simulink model "SporadicImpulse_6DOF"  (R2019a)
settings: Solver=VariableStepAuto  StartTime=0.0  StopTime=40  RelTol=1e-3
InitFcn:
  | Sporadic_Impulse_6DOF_init
values from neighbouring files (symbols this model uses):
  alpha_0 = 0    [Sporadic_Impulse_3DOF_init.m]    (also in Sporadic_Impulse_6DOF_init.m)
  beta_0 = 0    [Sporadic_Impulse_6DOF_init.m]
  g = 9.81    [Sporadic_Impulse_3DOF_init.m]    (also in Sporadic_Impulse_6DOF_init.m)
  gamma_0 = pi/2-deg2rad(6)    [Sporadic_Impulse_3DOF_init.m]    (also in Sporadic_Impulse_6DOF_init.m)
  m_0 = 40    [Sporadic_Impulse_3DOF_init.m]    (also in Sporadic_Impulse_6DOF_init.m)
  V_0 = 0.1    [Sporadic_Impulse_3DOF_init.m]    (also in Sporadic_Impulse_6DOF_init.m)
undefined symbols (not defined in the file or in its folder): F, Light, MIL
libraries: simulink_extras x4, aerolibwind2 x2, aerolibasang x1, aerolibatmos2 x1, vrlib x1, aerolib6dof2 x1, aerolibtransform2 x1
settings Model: Creator=Devansh  LastModifiedBy=Devansh

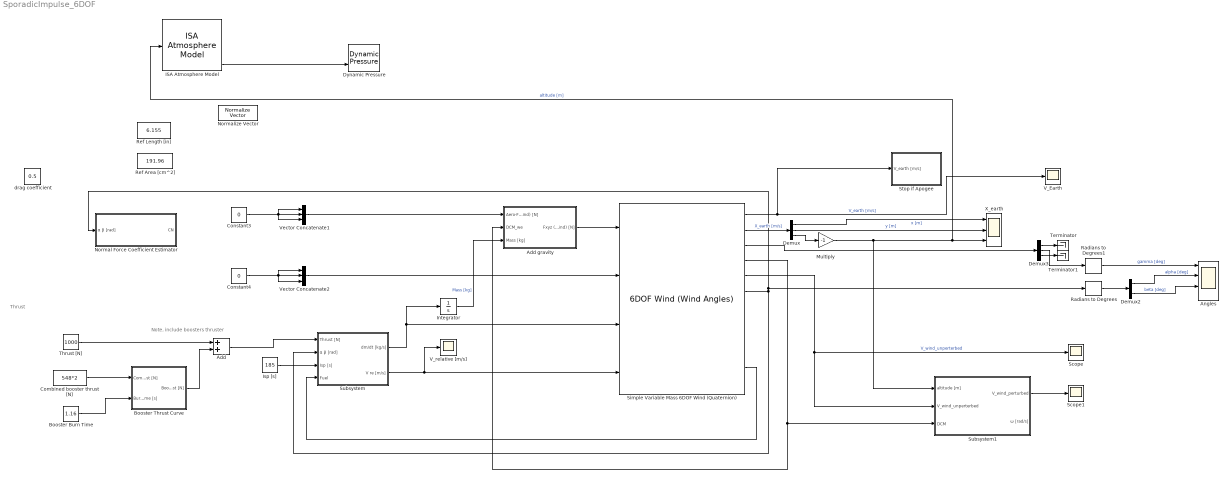
== system SporadicImpulse_6DOF ==
  note: Thrust
  note: Note, include boosters thruster
  Add : Sum
  Add gravity : Subsystem
  Angles : Scope  NumInputPorts=4
  Booster Burn Time : Constant  Value=1.16
  Booster Thrust Curve : Subsystem
  Combined booster thrust [N] : Constant  Value=548*2
  Constant3 : Constant  Value=0
  Constant4 : Constant  Value=0
  Demux : Demux  Outputs=3
  Demux2 : Demux  Outputs=2
  Demux3 : Demux  Outputs=3
  Dynamic Pressure : aerolibasang/Dynamic Pressure
  ISA Atmosphere Model : aerolibatmos2/ISA Atmosphere Model  custom=on  g=9.80665  gamma=1.4  R=287.0531  L=0.0065  h_trop=11000  h_strat=20000  rho0=1.225  P0=101325  T0=288.15  h0=0
      settings: SourceProductName=Aerospace Blockset
  Integrator : Integrator  InitialCondition=m_0
  Isp [s] : Constant  Value=185
  Multiply : Gain  Gain=-1
  Normal Force Coefficient Estimator : Subsystem
  Normalize Vector : vrlib/Utilities/Normalize Vector  maxzero=0
      settings: SourceProductName=Simulink
  Radians to Degrees : simulink_extras/Transformations/Radians to Degrees
  Radians to Degrees1 : simulink_extras/Transformations/Radians to Degrees
  Ref Area [cm^2] : Constant  Value=191.96
  Ref Length [in] : Constant  Value=6.155
  Scope : Scope
  Scope1 : Scope
  Simple Variable Mass 6DOF Wind (Quaternion) : aerolib6dof2/6DOF Wind (Wind Angles)  units=Metric (MKS)  mtype=Simple Variable  rep=Quaternion  xme_0=[0 0 0]  Vm_0=[V_0 alpha_0 beta_0]  wind_0=[0 gamma_0 0]  pm_0=[0 0 0]  mass_0=m_0  mass_e=m_dry  mass_f=m_0  inertia=eye(3)  inertia_e=I_dry  inertia_f=I_0  vre_flag=on  abi_flag=on  xme_statename=''  Vm_statename=''  alpha_statename=''  beta_statename=''  wind_statename=''  quat_statename=''  pm_statename=''  mass_statename=''
      settings: SourceProductName=Aerospace Blockset  SourceProductBaseCode=AE
  Stop if Apogee : Subsystem
  Subsystem : Subsystem
  Subsystem1 : Subsystem
  Terminator : Terminator
  Terminator1 : Terminator
  Thrust [N] : Constant  Value=1000
  V_Earth : Scope
  V_relative [m/s] : Scope
  Vector Concatenate1 : Concatenate  NumInputs=3
  Vector Concatenate2 : Concatenate  NumInputs=3
  X_earth : Scope  NumInputPorts=3
  drag coefficient : Constant  Value=0.5
  wires:
  Constant3/1 -> Vector Concatenate1/3, Vector Concatenate1/1, Vector Concatenate1/2
  Constant4/1 -> Vector Concatenate2/3, Vector Concatenate2/1, Vector Concatenate2/2
  Vector Concatenate2/1 -> Simple Variable Mass 6DOF Wind (Quaternion)/2
  Isp [s]/1 -> Subsystem/3(Isp [s])
  Vector Concatenate1/1 -> Add gravity/1(Aero-Forces (Wind) [N])
  Simple Variable Mass 6DOF Wind (Quaternion)/4 -> Add gravity/2(DCM_we), Subsystem1/3(DCM)
  Integrator/1 -> Add gravity/3(Mass [kg])  "Mass [kg]"
  Add gravity/1(Fxyz (Wind) [N]) -> Simple Variable Mass 6DOF Wind (Quaternion)/1
  Subsystem/1(dm/dt [kg/s]) -> Simple Variable Mass 6DOF Wind (Quaternion)/3, Integrator/1
  Simple Variable Mass 6DOF Wind (Quaternion)/11 -> Subsystem/4(Fuel)
  Simple Variable Mass 6DOF Wind (Quaternion)/1 -> Stop if Apogee/1(V_earth [m/s]), V_Earth/1  "V_earth [m/s]"
  Subsystem/2(V re [m/s]) -> Simple Variable Mass 6DOF Wind (Quaternion)/4, V_relative [m/s]/1
  Simple Variable Mass 6DOF Wind (Quaternion)/2 -> Demux/1  "X_earth [m/s]"
  Demux/3 -> Multiply/1
  Demux/1 -> X_earth/1  "x [m]"
  Demux/2 -> X_earth/2  "y [m]"
  Multiply/1 -> Subsystem1/1(altitude [m]), ISA Atmosphere Model/1, X_earth/3  "altitude [m]"
  Radians to Degrees/1 -> Demux2/1
  Demux2/1 -> Angles/2  "alpha [deg]"
  Demux2/2 -> Angles/3  "beta [deg]"
  Simple Variable Mass 6DOF Wind (Quaternion)/3 -> Demux3/1
  Demux3/2 -> Radians to Degrees1/1
  Thrust [N]/1 -> Add/1
  Add/1 -> Subsystem/1(Thrust [N])
  Combined booster thrust [N]/1 -> Booster Thrust Curve/1(Combined Thrust [N])
  Booster Burn Time/1 -> Booster Thrust Curve/2(Burn Time [s])
  Booster Thrust Curve/1(Booster Thrust [N]) -> Add/2
  Simple Variable Mass 6DOF Wind (Quaternion)/5 -> Scope/1, Subsystem1/2(V_wind_unperterbed)  "V_wind_unperterbed"
  Simple Variable Mass 6DOF Wind (Quaternion)/6 -> Radians to Degrees/1, Normal Force Coefficient Estimator/1(α β [rad]), Subsystem/2(α β [rad])
  ISA Atmosphere Model/4 -> Dynamic Pressure/2
  Demux3/1 -> Terminator/1
  Demux3/3 -> Terminator1/1
  Radians to Degrees1/1 -> Angles/1  "gamma [deg]"
  Subsystem1/1(V_wind_perturbed) -> Scope1/1

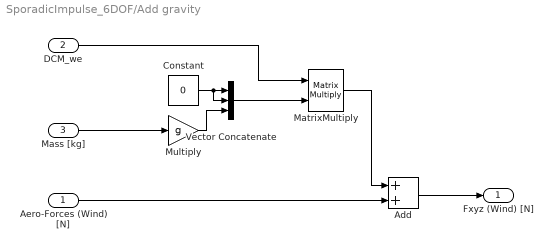
== system SporadicImpulse_6DOF/Add gravity ==
  Aero-Forces (Wind) [N] : Inport
  DCM_we : Inport  Port=2
  Mass [kg] : Inport  Port=3
  Add : Sum
  Constant : Constant  Value=0
  MatrixMultiply : Product  Multiplication=Matrix(*)
  Multiply : Gain  Gain=g
  Vector Concatenate : Concatenate  NumInputs=3
  Fxyz (Wind) [N] : Outport
  wires:
  Aero-Forces (Wind) [N]/1 -> Add/2
  MatrixMultiply/1 -> Add/1
  DCM_we/1 -> MatrixMultiply/1
  Mass [kg]/1 -> Multiply/1
  Multiply/1 -> Vector Concatenate/3
  Constant/1 -> Vector Concatenate/1, Vector Concatenate/2
  Vector Concatenate/1 -> MatrixMultiply/2
  Add/1 -> Fxyz (Wind) [N]/1

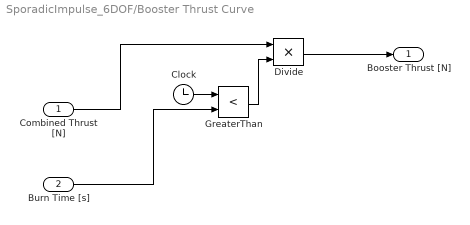
== system SporadicImpulse_6DOF/Booster Thrust Curve ==
  Combined Thrust [N] : Inport
  Burn Time [s] : Inport  Port=2
  Clock : Clock
  Divide : Product  Inputs=**
  GreaterThan : RelationalOperator  Operator=<  OutDataTypeStr=boolean  RndMeth=Simplest
  Booster Thrust [N] : Outport
  wires:
  Combined Thrust [N]/1 -> Divide/1
  Clock/1 -> GreaterThan/1
  Divide/1 -> Booster Thrust [N]/1
  Burn Time [s]/1 -> GreaterThan/2
  GreaterThan/1 -> Divide/2

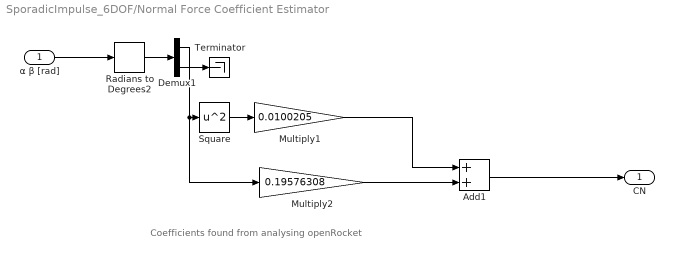
== system SporadicImpulse_6DOF/Normal Force Coefficient Estimator ==
  note: Coefficients found from analysing openRocket
  α β [rad] : Inport
  Add1 : Sum
  Demux1 : Demux  Outputs=2
  Multiply1 : Gain  Gain=0.0100205
  Multiply2 : Gain  Gain=0.19576308
  Radians to Degrees2 : simulink_extras/Transformations/Radians to Degrees
  Square : Math  Operator=square  SaturateOnIntegerOverflow=on
  Terminator : Terminator
  CN : Outport
  wires:
  Add1/1 -> CN/1
  α β [rad]/1 -> Radians to Degrees2/1
  Radians to Degrees2/1 -> Demux1/1
  Demux1/1 -> Multiply2/1, Square/1
  Demux1/2 -> Terminator/1
  Square/1 -> Multiply1/1
  Multiply1/1 -> Add1/1
  Multiply2/1 -> Add1/2

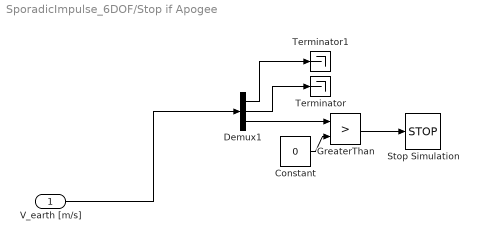
== system SporadicImpulse_6DOF/Stop if Apogee ==
  V_earth [m/s] : Inport
  Constant : Constant  Value=0
  Demux1 : Demux  Outputs=3
  GreaterThan : RelationalOperator  Operator=>  OutDataTypeStr=boolean  RndMeth=Simplest
  Stop Simulation : Stop
  Terminator : Terminator
  Terminator1 : Terminator
  wires:
  Demux1/1 -> Terminator1/1
  Constant/1 -> GreaterThan/2
  Demux1/2 -> Terminator/1
  Demux1/3 -> GreaterThan/1
  V_earth [m/s]/1 -> Demux1/1
  GreaterThan/1 -> Stop Simulation/1

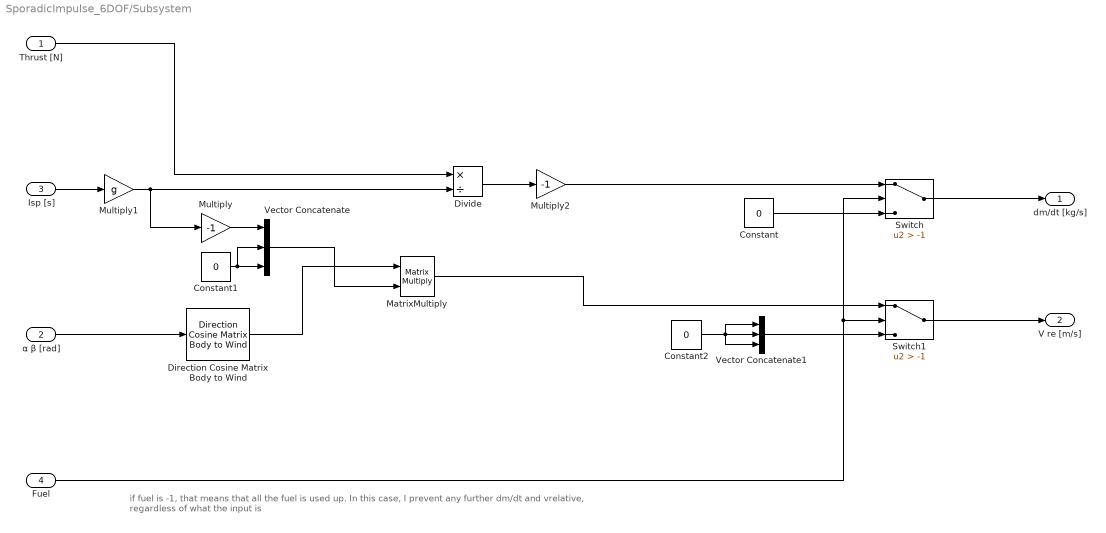
== system SporadicImpulse_6DOF/Subsystem ==
  note: if fuel is -1, that means that all the fuel is used up. In this case, I prevent any further dm/dt and vrelative, regardless of what the input is
  Thrust [N] : Inport
  α β [rad] : Inport  Port=2
  Isp [s] : Inport  Port=3
  Fuel : Inport  Port=4
  Constant : Constant  Value=0
  Constant1 : Constant  Value=0
  Constant2 : Constant  Value=0
  Direction Cosine Matrix Body to Wind : aerolibtransform2/Direction Cosine Matrix Body to Wind
      settings: SourceProductName=Aerospace Blockset  SourceProductBaseCode=AE
  Divide : Product  Inputs=*/
  MatrixMultiply : Product  Multiplication=Matrix(*)
  Multiply : Gain  Gain=-1
  Multiply1 : Gain  Gain=g
  Multiply2 : Gain  Gain=-1
  Switch : Switch  Criteria=u2 > Threshold  Threshold=-1
  Switch1 : Switch  Criteria=u2 > Threshold  Threshold=-1
  Vector Concatenate : Concatenate  NumInputs=3
  Vector Concatenate1 : Concatenate  NumInputs=3
  dm/dt [kg/s] : Outport
  V re [m/s] : Outport  Port=2
  wires:
  α β [rad]/1 -> Direction Cosine Matrix Body to Wind/1
  Divide/1 -> Multiply2/1
  Multiply/1 -> Vector Concatenate/1
  Isp [s]/1 -> Multiply1/1
  Direction Cosine Matrix Body to Wind/1 -> MatrixMultiply/1
  Constant1/1 -> Vector Concatenate/2, Vector Concatenate/3
  Vector Concatenate/1 -> MatrixMultiply/2
  Thrust [N]/1 -> Divide/1
  Multiply1/1 -> Multiply/1, Divide/2
  Fuel/1 -> Switch1/2, Switch/2
  Switch/1 -> dm/dt [kg/s]/1
  Multiply2/1 -> Switch/1
  Constant/1 -> Switch/3
  Switch1/1 -> V re [m/s]/1
  MatrixMultiply/1 -> Switch1/1
  Constant2/1 -> Vector Concatenate1/3, Vector Concatenate1/2, Vector Concatenate1/1
  Vector Concatenate1/1 -> Switch1/3

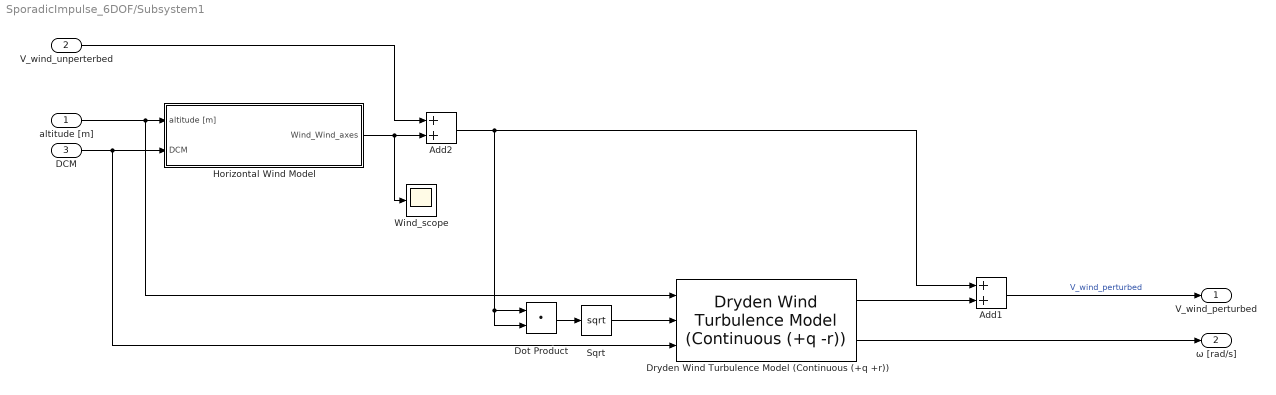
== system SporadicImpulse_6DOF/Subsystem1 ==
  altitude [m] : Inport
  V_wind_unperterbed : Inport  Port=2
  DCM : Inport  Port=3
  Add1 : Sum
  Add2 : Sum
  Dot Product : DotProduct  InputSameDT=on  OutDataTypeStr=Inherit: Inherit via internal rule
  Dryden Wind Turbulence Model (Continuous (+q +r)) : aerolibwind2/Dryden Wind Turbulence Model  (Continuous (+q -r))  units=Metric (MKS)  spec=MIL-F-8785C  model=Continuous Dryden (+q -r)  W20=10  Wdeg=0  TurbProb=10^-2 - Light  L_high=533.4  Wingspan=4  ts=0.1  Seed=[23341 23342 23343 23344]  T_on=on
      settings: SourceProductName=Aerospace Blockset
  Horizontal Wind Model : Subsystem
  Sqrt : Sqrt  SaturateOnIntegerOverflow=on
  Wind_scope : Scope
  V_wind_perturbed : Outport
  ω [rad/s] : Outport  Port=2
  wires:
  Add1/1 -> V_wind_perturbed/1  "V_wind_perturbed"
  V_wind_unperterbed/1 -> Add2/1
  DCM/1 -> Dryden Wind Turbulence Model (Continuous (+q +r))/3, Horizontal Wind Model/2(DCM)
  Dryden Wind Turbulence Model (Continuous (+q +r))/1 -> Add1/2
  Dryden Wind Turbulence Model (Continuous (+q +r))/2 -> ω [rad/s]/1
  altitude [m]/1 -> Dryden Wind Turbulence Model (Continuous (+q +r))/1, Horizontal Wind Model/1(altitude [m])
  Horizontal Wind Model/1(Wind_Wind_axes) -> Wind_scope/1, Add2/2
  Add2/1 -> Dot Product/2, Dot Product/1, Add1/1
  Dot Product/1 -> Sqrt/1
  Sqrt/1 -> Dryden Wind Turbulence Model (Continuous (+q +r))/2

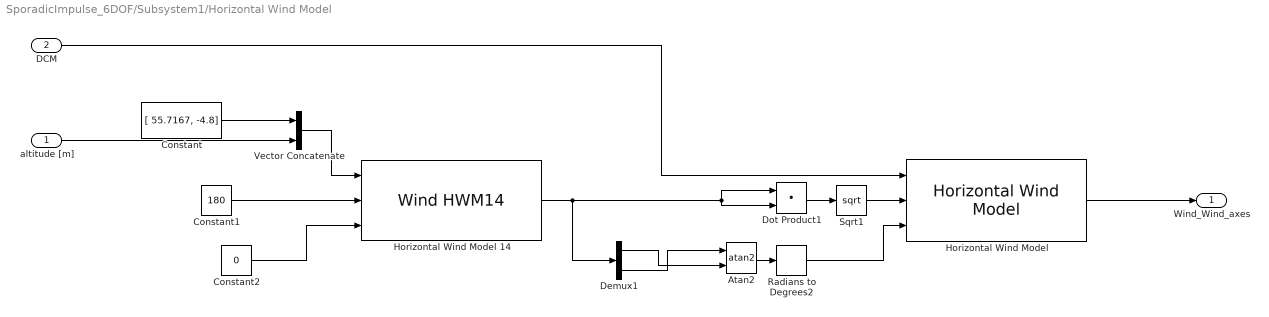
== system SporadicImpulse_6DOF/Subsystem1/Horizontal Wind Model ==
  altitude [m] : Inport
  DCM : Inport  Port=2
  Atan2 : Trigonometry  Operator=atan2
  Constant : Constant  Value=[ 55.7167, -4.8]
  Constant1 : Constant  Value=180
  Constant2 : Constant  Value=0
  Demux1 : Demux  Outputs=2
  Dot Product1 : DotProduct  InputSameDT=on  OutDataTypeStr=Inherit: Inherit via internal rule
  Horizontal Wind Model : aerolibwind2/Horizontal Wind Model  units=Metric (MKS)  Vw_source=External  Vwind=15  W_source=External  Wdeg=0
      settings: SourceProductName=Aerospace Blockset  SourceProductBaseCode=AE
  Horizontal Wind Model 14 : WindHWM14
  Radians to Degrees2 : simulink_extras/Transformations/Radians to Degrees
  Sqrt1 : Sqrt  SaturateOnIntegerOverflow=on
  Vector Concatenate : Concatenate
  Wind_Wind_axes : Outport
  wires:
  Horizontal Wind Model/1 -> Wind_Wind_axes/1
  Constant1/1 -> Horizontal Wind Model 14/2
  Constant2/1 -> Horizontal Wind Model 14/3
  altitude [m]/1 -> Vector Concatenate/2
  Demux1/2 -> Atan2/1
  Horizontal Wind Model 14/1 -> Dot Product1/1, Dot Product1/2, Demux1/1
  Dot Product1/1 -> Sqrt1/1
  Sqrt1/1 -> Horizontal Wind Model/2
  Constant/1 -> Vector Concatenate/1
  Atan2/1 -> Radians to Degrees2/1
  Vector Concatenate/1 -> Horizontal Wind Model 14/1
  Radians to Degrees2/1 -> Horizontal Wind Model/3
  DCM/1 -> Horizontal Wind Model/1
  Demux1/1 -> Atan2/2
